simulink model "adaptivePID"  (R2024a)
settings: Solver=ode4  StartTime=0.0  StopTime=5  FixedStep=1E-5  RelTol=1e-3
values from neighbouring files (symbols this model uses):
  initial_1 =     [ma.mat]    (also in regulation.mat)
  observer =     [ma.mat]    (also in regulation.mat)
  sliding =     [regulation.mat]
  x = [input(1);input(2);input(3)]    [Dist_observer.m]    (also in is501nmtbModel_simu.m; is501nmtbModel_simu1.m; ma.mat = ; neuronalPID.m = entr(4))
  y = [input(7),input(8),input(9)]'    [estimator.m]    (also in is501nmtbModel_simu1.m = B * x + Td; ma.mat = ; regulation.mat = )
  z =     [ma.mat]    (also in regulation.mat)
settings Model: Creator=b_ant  LastModifiedBy=b_ant
settings SolverCC: ZeroCrossAlgorithm=Adaptive
settings DebuggingCC: IgnoredZcDiagnostic=none  UnconnectedInputMsg=warning  UnconnectedOutputMsg=warning  UnconnectedLineMsg=warning
settings ModelReferenceCC: EnableRefExpFcnMdlSchedulingChecks=on
settings RTWCC: GPUComputeCapability=3.5  DLArmComputeVersion=19.05

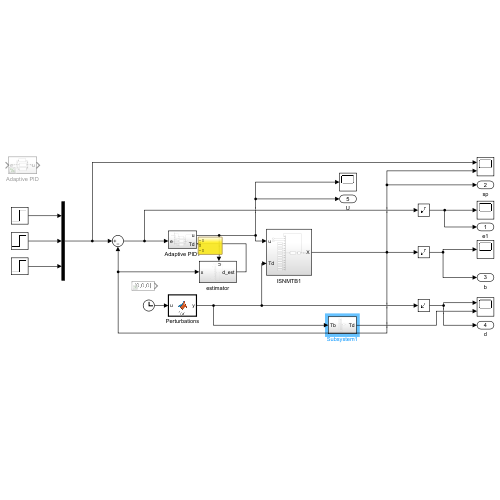
[thumbnail: Simulink's stored preview of the top-level diagram]
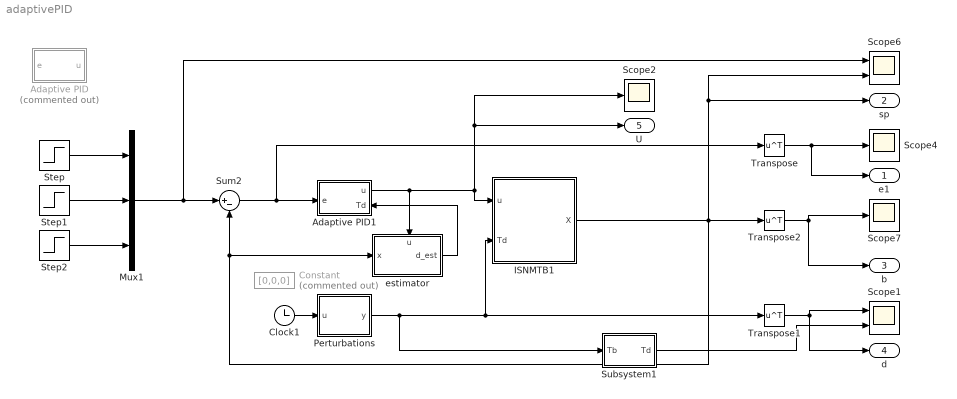
== system adaptivePID ==
  Adaptive PID : Subsystem  Commented=on
  Adaptive PID1 : Subsystem
      settings: PortSchema="{\"entries\":[{\"content\":{\"sides\":[{\"content\":{\"connectorIds\":[\"In1\"]},\"type\":\"ConnectorPlacement.EquallySpacedRectSide\",\"uuid\":\"d8958802-6b7a-44a5-a52a-ddab063e146c\"},{\"content\":{\"connectorIds\":[\"Out1\",\"In2\"],\"side\":\"RIGHT\"},\"type\":\"ConnectorPlacement.EquallySpacedRectSide\",\"uuid\":\"da9beaf8-944d-47f3-af69-928c263140b5\"},{\"content\":{\"side\":\"TOP\"},\"type\":\"ConnectorPlacement.EquallySpacedRectSide\",\"uuid\":\"6b1d50a8-02e3-44c8-b40e-0b40ffb17dcd\"}]},\"type\":\"ConnectorPlacement.EquallySpacedConnector\",\"uuid\":\"8706e551-040c-4dd8-82c5-a7bc820e0e37\"}],\"packageUris\":[\"http://schema.mathworks.com/mf0/Connector/R2020b\"],\"version\":\"1.0\"}"
  Clock1 : Clock
      settings: Decimation=1000
  Constant : Constant  Commented=on  Value=[0,0,0]
  ISNMTB1 : Subsystem
  Mux1 : Mux  Inputs=3
  Perturbations : MATLAB Function  TreatAsAtomicUnit=on
  Scope1 : Scope  NumInputPorts=2
  Scope2 : Scope
  Scope4 : Scope
  Scope6 : Scope  NumInputPorts=2
  Scope7 : Scope
  Step : Step  Time=0.1  SampleTime=0
  Step1 : Step  Time=0.1  SampleTime=0
  Step2 : Step  Time=0.1  After=0.1  SampleTime=0
  Subsystem1 : Subsystem
  Sum2 : Sum  Inputs=|+-
  Transpose : Math  Operator=transpose
  Transpose1 : Math  Operator=transpose
  Transpose2 : Math  Operator=transpose
  estimator : Subsystem
      settings: PortSchema="{\"entries\":[{\"content\":{\"sides\":[{\"content\":{\"connectorIds\":[\"In1\"]},\"type\":\"ConnectorPlacement.EquallySpacedRectSide\",\"uuid\":\"f9e844d6-ee13-4ae8-8d73-084dc6b9c230\"},{\"content\":{\"connectorIds\":[\"Out1\"],\"side\":\"RIGHT\"},\"type\":\"ConnectorPlacement.EquallySpacedRectSide\",\"uuid\":\"c081e574-2129-4344-8b67-56cd55c23b50\"},{\"content\":{\"connectorIds\":[\"In2\"],\"side\":\"TOP\"},\"type\":\"ConnectorPlacement.EquallySpacedRectSide\",\"uuid\":\"bf6f2985-e51e-41d0-a8b1-b5505659e5f3\"},{\"content\":{\"side\":\"BOTTOM\"},\"type\":\"ConnectorPlacement.EquallySpacedRectSide\",\"uuid\":\"e1697b77-960b-449d-843b-5909cf972339\"}]},\"type\":\"ConnectorPlacement.EquallySpacedConnector\",\"uuid\":\"c9da1c41-5311-41bf-ab5b-06506202d90f\"}],\"packageUris\":[\"http://schema.mathworks.com/mf0/Connector/R2020b\"],\"version\":\"1.0\"}"
  e1 : Outport
  sp : Outport  Port=2
  b : Outport  Port=3
  d : Outport  Port=4
  U : Outport  Port=5
  wires:
  Transpose1/1 -> Scope1/1, d/1
  ISNMTB1/1(X) -> sp/1, Scope6/2, estimator/1(x), Sum2/2, Transpose2/1
  Sum2/1 -> Transpose/1, Adaptive PID1/1(e)
  Step2/1 -> Mux1/3
  Transpose2/1 -> Scope7/1, b/1
  Step1/1 -> Mux1/2
  Clock1/1 -> Perturbations/1(u)
  Transpose/1 -> e1/1, Scope4/1
  Step/1 -> Mux1/1
  Mux1/1 -> Sum2/1, Scope6/1
  Adaptive PID1/1(u) -> estimator/2(u), ISNMTB1/1(u), U/1, Scope2/1
  estimator/1(d_est) -> Adaptive PID1/2(Td)
  Subsystem1/1(Td) -> Scope1/2
  Perturbations/1(y) -> ISNMTB1/2(Td), Transpose1/1, Subsystem1/1(Tb)

== system adaptivePID/Adaptive PID ==
  e : Inport
  Demux1 : Demux  Outputs=3
  Mux : Mux  Inputs=3
  x controller : Subsystem
  y controller : Subsystem
  z controller : Subsystem
  u : Outport
  wires:
  z controller/1(u) -> Mux/3
  Demux1/2 -> y controller/1(e)
  x controller/1(u) -> Mux/1
  e/1 -> Demux1/1
  y controller/1(u) -> Mux/2
  Demux1/3 -> z controller/1(e)
  Demux1/1 -> x controller/1(e)
  Mux/1 -> u/1

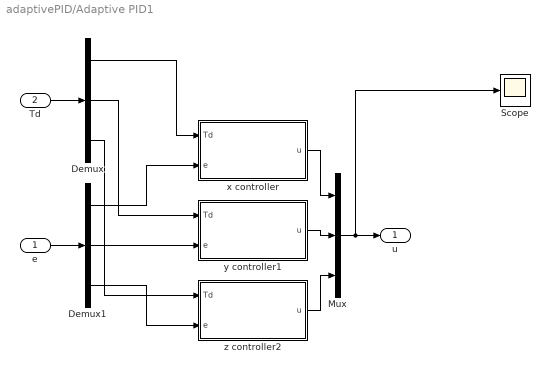
== system adaptivePID/Adaptive PID1 ==
  e : Inport
  Td : Inport  Port=2
  Demux : Demux  Outputs=3
  Demux1 : Demux  Outputs=3
  Mux : Mux  Inputs=3
  Scope : Scope
  x controller : Subsystem
  y controller1 : Subsystem
  z controller2 : Subsystem
  u : Outport
  wires:
  Demux1/2 -> y controller1/2(e)
  x controller/1(u) -> Mux/1
  e/1 -> Demux1/1
  Demux1/1 -> x controller/2(e)
  Mux/1 -> Scope/1, u/1
  Demux1/3 -> z controller2/2(e)
  Demux/3 -> z controller2/1(Td)
  Demux/2 -> y controller1/1(Td)
  Demux/1 -> x controller/1(Td)
  Td/1 -> Demux/1
  y controller1/1(u) -> Mux/2
  z controller2/1(u) -> Mux/3

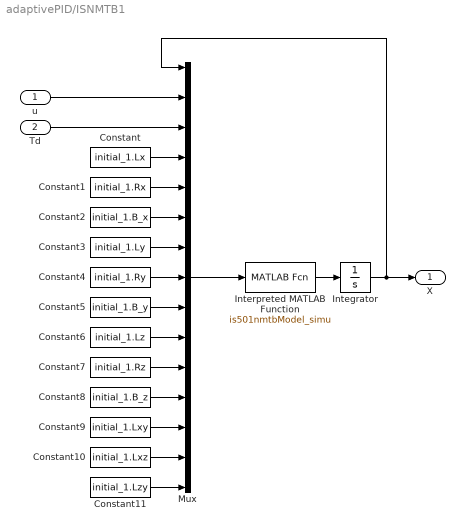
== system adaptivePID/ISNMTB1 ==
  u : Inport
  Td : Inport  Port=2
  Constant : Constant  Value=initial_1.Lx
  Constant1 : Constant  Value=initial_1.Rx
  Constant10 : Constant  Value=initial_1.Lxz
  Constant11 : Constant  Value=initial_1.Lzy
  Constant2 : Constant  Value=initial_1.B_x
  Constant3 : Constant  Value=initial_1.Ly
  Constant4 : Constant  Value=initial_1.Ry
  Constant5 : Constant  Value=initial_1.B_y
  Constant6 : Constant  Value=initial_1.Lz
  Constant7 : Constant  Value=initial_1.Rz
  Constant8 : Constant  Value=initial_1.B_z
  Constant9 : Constant  Value=initial_1.Lxy
  Integrator : Integrator  InitialCondition=[3.249E4, -2.265E4, 3.655E4]
  Interpreted MATLAB Function : MATLABFcn  MATLABFcn=is501nmtbModel_simu
  Mux : Mux  Inputs=15
  X : Outport
  wires:
  Interpreted MATLAB Function/1 -> Integrator/1
  Integrator/1 -> X/1, Mux/1
  Mux/1 -> Interpreted MATLAB Function/1
  u/1 -> Mux/2
  Td/1 -> Mux/3
  Constant/1 -> Mux/4
  Constant1/1 -> Mux/5
  Constant2/1 -> Mux/6
  Constant3/1 -> Mux/7
  Constant4/1 -> Mux/8
  Constant5/1 -> Mux/9
  Constant6/1 -> Mux/10
  Constant7/1 -> Mux/11
  Constant8/1 -> Mux/12
  Constant9/1 -> Mux/13
  Constant10/1 -> Mux/14
  Constant11/1 -> Mux/15

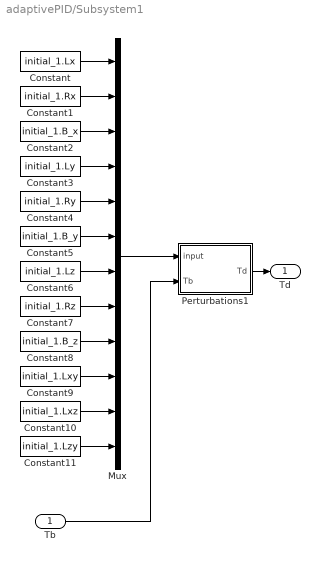
== system adaptivePID/Subsystem1 ==
  Tb : Inport
  Constant : Constant  Value=initial_1.Lx
  Constant1 : Constant  Value=initial_1.Rx
  Constant10 : Constant  Value=initial_1.Lxz
  Constant11 : Constant  Value=initial_1.Lzy
  Constant2 : Constant  Value=initial_1.B_x
  Constant3 : Constant  Value=initial_1.Ly
  Constant4 : Constant  Value=initial_1.Ry
  Constant5 : Constant  Value=initial_1.B_y
  Constant6 : Constant  Value=initial_1.Lz
  Constant7 : Constant  Value=initial_1.Rz
  Constant8 : Constant  Value=initial_1.B_z
  Constant9 : Constant  Value=initial_1.Lxy
  Mux : Mux  Inputs=12
  Perturbations1 : MATLAB Function  TreatAsAtomicUnit=on
  Td : Outport
  wires:
  Constant2/1 -> Mux/3
  Constant6/1 -> Mux/7
  Constant7/1 -> Mux/8
  Constant8/1 -> Mux/9
  Constant9/1 -> Mux/10
  Constant/1 -> Mux/1
  Constant11/1 -> Mux/12
  Constant10/1 -> Mux/11
  Constant5/1 -> Mux/6
  Constant3/1 -> Mux/4
  Mux/1 -> Perturbations1/1(input)
  Constant1/1 -> Mux/2
  Constant4/1 -> Mux/5
  Tb/1 -> Perturbations1/2(Tb)
  Perturbations1/1(Td) -> Td/1

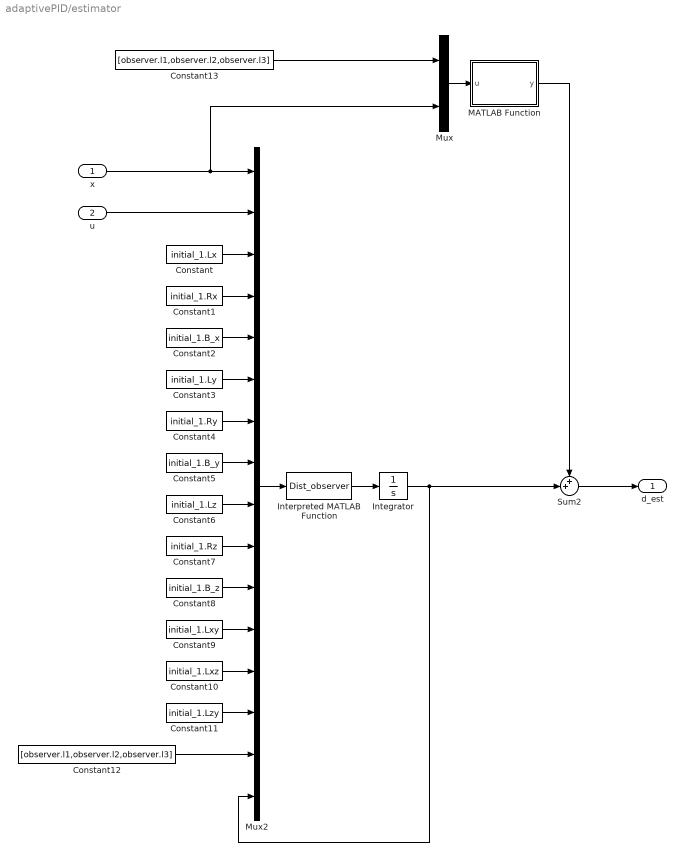
== system adaptivePID/estimator ==
  x : Inport
  u : Inport  Port=2
  Constant : Constant  Value=initial_1.Lx
  Constant1 : Constant  Value=initial_1.Rx
  Constant10 : Constant  Value=initial_1.Lxz
  Constant11 : Constant  Value=initial_1.Lzy
  Constant12 : Constant  Value=[observer.l1,observer.l2,observer.l3]
  Constant13 : Constant  Value=[observer.l1,observer.l2,observer.l3]
  Constant2 : Constant  Value=initial_1.B_x
  Constant3 : Constant  Value=initial_1.Ly
  Constant4 : Constant  Value=initial_1.Ry
  Constant5 : Constant  Value=initial_1.B_y
  Constant6 : Constant  Value=initial_1.Lz
  Constant7 : Constant  Value=initial_1.Rz
  Constant8 : Constant  Value=initial_1.B_z
  Constant9 : Constant  Value=initial_1.Lxy
  Integrator : Integrator  InitialCondition=[0,0,0]
  Interpreted MATLAB Function : MATLABFcn  MATLABFcn=Dist_observer
  MATLAB Function : MATLAB Function  TreatAsAtomicUnit=on
  Mux : Mux  Inputs=2
  Mux2 : Mux  Inputs=16
  Sum2 : Sum  Inputs=++|
  d_est : Outport
  wires:
  Constant6/1 -> Mux2/9
  MATLAB Function/1(y) -> Sum2/1
  Constant10/1 -> Mux2/13
  Integrator/1 -> Sum2/2, Mux2/16
  Interpreted MATLAB Function/1 -> Integrator/1
  Constant2/1 -> Mux2/5
  Constant4/1 -> Mux2/7
  Constant7/1 -> Mux2/10
  Mux2/1 -> Interpreted MATLAB Function/1
  Constant11/1 -> Mux2/14
  Constant8/1 -> Mux2/11
  Constant1/1 -> Mux2/4
  Constant3/1 -> Mux2/6
  Constant/1 -> Mux2/3
  Constant9/1 -> Mux2/12
  Constant5/1 -> Mux2/8
  Constant12/1 -> Mux2/15
  u/1 -> Mux2/2
  Sum2/1 -> d_est/1
  Constant13/1 -> Mux/1
  Mux/1 -> MATLAB Function/1(u)
  x/1 -> Mux/2, Mux2/1

== system adaptivePID/Adaptive PID/x controller ==
  e : Inport
  Adaptation Law : Subsystem  mask{alpha=x.alpha, beta=x.beta, epsilon=x.epsilon, n=x.n, kd0=x.kd_init, ki0=x.ki_init, kp0=x.kp_init}
      mask prompts: kd0 "kd_0:"; ki0 "ki_0:"; kp0 "kp_0:"
      mask TypeOptions alpha: alpha/Value
      mask TypeOptions beta: beta/Value
      mask TypeOptions epsilon: epsilon/Value
      mask TypeOptions n: n/Value
      mask TypeOptions kd0: kd0/Value
      mask TypeOptions ki0: ki0/Value
      mask TypeOptions kp0: kp0/Value
  PID controller : Subsystem
  Scope : Scope
  Sliding surface : Subsystem  mask{Gain=x.lambda}
      mask prompts: Gain "Simulink:blkprm_prompts:GainGain"
      mask TypeOptions Gain: Gain/Gain
      mask DialogControl Gain Prompt: Gain:
  error subsystem : Subsystem
  u : Outport
  wires:
  Sliding surface/1(s) -> Adaptation Law/2(s)
  Sliding surface/2(s_dot) -> Adaptation Law/3(s_dot)
  PID controller/1(u) -> u/1
  error subsystem/1(MyPi) -> PID controller/2(MyPi), Adaptation Law/1(myPi)
  e/1 -> Sliding surface/1(e), error subsystem/1(e)
  Adaptation Law/1(theta) -> Scope/1, PID controller/1(theta)

== system adaptivePID/Adaptive PID/y controller ==
  e : Inport
  Adaptation Law : Subsystem  mask{alpha=y.alpha, beta=y.beta, epsilon=y.epsilon, n=y.n, kd0=y.kd_init, ki0=y.ki_init, kp0=y.kp_init}
      mask prompts: kd0 "kd_0:"; ki0 "ki_0:"; kp0 "kp_0:"
      mask TypeOptions alpha: alpha/Value
      mask TypeOptions beta: beta/Value
      mask TypeOptions epsilon: epsilon/Value
      mask TypeOptions n: n/Value
      mask TypeOptions kd0: kd0/Value
      mask TypeOptions ki0: ki0/Value
      mask TypeOptions kp0: kp0/Value
  PID controller : Subsystem
  Scope : Scope
  Sliding surface : Subsystem  mask{Gain=y.lambda}
      mask prompts: Gain "Simulink:blkprm_prompts:GainGain"
      mask TypeOptions Gain: Gain/Gain
      mask DialogControl Gain Prompt: Gain:
  error subsystem : Subsystem
  u : Outport
  wires:
  e/1 -> Sliding surface/1(e), error subsystem/1(e)
  error subsystem/1(MyPi) -> Adaptation Law/1(myPi), PID controller/2(MyPi)
  Adaptation Law/1(theta) -> PID controller/1(theta), Scope/1
  PID controller/1(u) -> u/1
  Sliding surface/2(s_dot) -> Adaptation Law/3(s_dot)
  Sliding surface/1(s) -> Adaptation Law/2(s)

== system adaptivePID/Adaptive PID/z controller ==
  e : Inport
  Adaptation Law : Subsystem  mask{alpha=z.alpha, beta=z.beta, epsilon=z.epsilon, n=z.n, kd0=z.kd_init, ki0=z.ki_init, kp0=z.kp_init}
      mask prompts: kd0 "kd_0:"; ki0 "ki_0:"; kp0 "kp_0:"
      mask TypeOptions alpha: alpha/Value
      mask TypeOptions beta: beta/Value
      mask TypeOptions epsilon: epsilon/Value
      mask TypeOptions n: n/Value
      mask TypeOptions kd0: kd0/Value
      mask TypeOptions ki0: ki0/Value
      mask TypeOptions kp0: kp0/Value
  PID controller : Subsystem
  Scope : Scope
  Sliding surface : Subsystem  mask{Gain=z.lambda}
      mask prompts: Gain "Simulink:blkprm_prompts:GainGain"
      mask TypeOptions Gain: Gain/Gain
      mask DialogControl Gain Prompt: Gain:
  error subsystem : Subsystem
  u : Outport
  wires:
  Sliding surface/1(s) -> Adaptation Law/2(s)
  Sliding surface/2(s_dot) -> Adaptation Law/3(s_dot)
  PID controller/1(u) -> u/1
  Adaptation Law/1(theta) -> Scope/1, PID controller/1(theta)
  error subsystem/1(MyPi) -> PID controller/2(MyPi), Adaptation Law/1(myPi)
  e/1 -> error subsystem/1(e), Sliding surface/1(e)

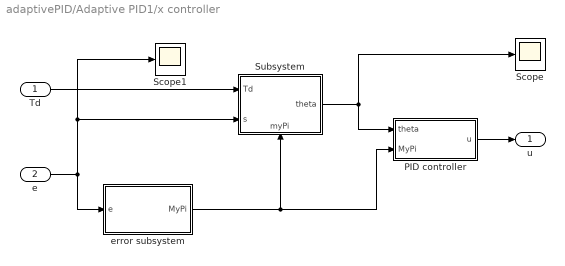
== system adaptivePID/Adaptive PID1/x controller ==
  Td : Inport
  e : Inport  Port=2
  PID controller : Subsystem
  Scope : Scope
  Scope1 : Scope
  Subsystem : Subsystem
      settings: PortSchema="{\"entries\":[{\"content\":{\"sides\":[{\"content\":{\"connectorIds\":[\"In1\",\"In2\"]},\"type\":\"ConnectorPlacement.EquallySpacedRectSide\",\"uuid\":\"240bad6f-f804-428c-a3a0-dcf6f9934484\"},{\"content\":{\"connectorIds\":[\"Out1\"],\"side\":\"RIGHT\"},\"type\":\"ConnectorPlacement.EquallySpacedRectSide\",\"uuid\":\"1a0c794f-cbf7-475a-a374-9465cebda297\"},{\"content\":{\"side\":\"TOP\"},\"type\":\"ConnectorPlacement.EquallySpacedRectSide\",\"uuid\":\"3b98e4f4-718b-47e5-85a1-a51970b349c9\"},{\"content\":{\"connectorIds\":[\"In3\"],\"side\":\"BOTTOM\"},\"type\":\"ConnectorPlacement.EquallySpacedRectSide\",\"uuid\":\"519e2597-1479-45b2-9e81-d744a6fccd79\"}]},\"type\":\"ConnectorPlacement.EquallySpacedConnector\",\"uuid\":\"08a721e1-b25b-470b-a637-c1c50488aa37\"}],\"packageUris\":[\"http://schema.mathworks.com/mf0/Connector/R2020b\"],\"version\":\"1.0\"}"
  error subsystem : Subsystem
  u : Outport
  wires:
  PID controller/1(u) -> u/1
  error subsystem/1(MyPi) -> Subsystem/3(myPi), PID controller/2(MyPi)
  e/1 -> error subsystem/1(e), Scope1/1, Subsystem/2(s)
  Subsystem/1(theta) -> Scope/1, PID controller/1(theta)
  Td/1 -> Subsystem/1(Td)

== system adaptivePID/Adaptive PID1/y controller1 ==
  Td : Inport
  e : Inport  Port=2
  PID controller : Subsystem
  Scope : Scope
  Subsystem : Subsystem
      settings: PortSchema="{\"entries\":[{\"content\":{\"sides\":[{\"content\":{\"connectorIds\":[\"In1\",\"In2\"]},\"type\":\"ConnectorPlacement.EquallySpacedRectSide\",\"uuid\":\"240bad6f-f804-428c-a3a0-dcf6f9934484\"},{\"content\":{\"connectorIds\":[\"Out1\"],\"side\":\"RIGHT\"},\"type\":\"ConnectorPlacement.EquallySpacedRectSide\",\"uuid\":\"1a0c794f-cbf7-475a-a374-9465cebda297\"},{\"content\":{\"side\":\"TOP\"},\"type\":\"ConnectorPlacement.EquallySpacedRectSide\",\"uuid\":\"3b98e4f4-718b-47e5-85a1-a51970b349c9\"},{\"content\":{\"connectorIds\":[\"In3\"],\"side\":\"BOTTOM\"},\"type\":\"ConnectorPlacement.EquallySpacedRectSide\",\"uuid\":\"519e2597-1479-45b2-9e81-d744a6fccd79\"}]},\"type\":\"ConnectorPlacement.EquallySpacedConnector\",\"uuid\":\"08a721e1-b25b-470b-a637-c1c50488aa37\"}],\"packageUris\":[\"http://schema.mathworks.com/mf0/Connector/R2020b\"],\"version\":\"1.0\"}"
  error subsystem : Subsystem
  u : Outport
  wires:
  PID controller/1(u) -> u/1
  error subsystem/1(MyPi) -> Subsystem/3(myPi), PID controller/2(MyPi)
  e/1 -> error subsystem/1(e), Subsystem/2(s)
  Subsystem/1(theta) -> Scope/1, PID controller/1(theta)
  Td/1 -> Subsystem/1(Td)

== system adaptivePID/Adaptive PID1/z controller2 ==
  Td : Inport
  e : Inport  Port=2
  PID controller : Subsystem
  Scope : Scope
  Subsystem : Subsystem
      settings: PortSchema="{\"entries\":[{\"content\":{\"sides\":[{\"content\":{\"connectorIds\":[\"In1\",\"In2\"]},\"type\":\"ConnectorPlacement.EquallySpacedRectSide\",\"uuid\":\"240bad6f-f804-428c-a3a0-dcf6f9934484\"},{\"content\":{\"connectorIds\":[\"Out1\"],\"side\":\"RIGHT\"},\"type\":\"ConnectorPlacement.EquallySpacedRectSide\",\"uuid\":\"1a0c794f-cbf7-475a-a374-9465cebda297\"},{\"content\":{\"side\":\"TOP\"},\"type\":\"ConnectorPlacement.EquallySpacedRectSide\",\"uuid\":\"3b98e4f4-718b-47e5-85a1-a51970b349c9\"},{\"content\":{\"connectorIds\":[\"In3\"],\"side\":\"BOTTOM\"},\"type\":\"ConnectorPlacement.EquallySpacedRectSide\",\"uuid\":\"519e2597-1479-45b2-9e81-d744a6fccd79\"}]},\"type\":\"ConnectorPlacement.EquallySpacedConnector\",\"uuid\":\"08a721e1-b25b-470b-a637-c1c50488aa37\"}],\"packageUris\":[\"http://schema.mathworks.com/mf0/Connector/R2020b\"],\"version\":\"1.0\"}"
  error subsystem : Subsystem
  u : Outport
  wires:
  PID controller/1(u) -> u/1
  error subsystem/1(MyPi) -> Subsystem/3(myPi), PID controller/2(MyPi)
  e/1 -> error subsystem/1(e), Subsystem/2(s)
  Subsystem/1(theta) -> Scope/1, PID controller/1(theta)
  Td/1 -> Subsystem/1(Td)

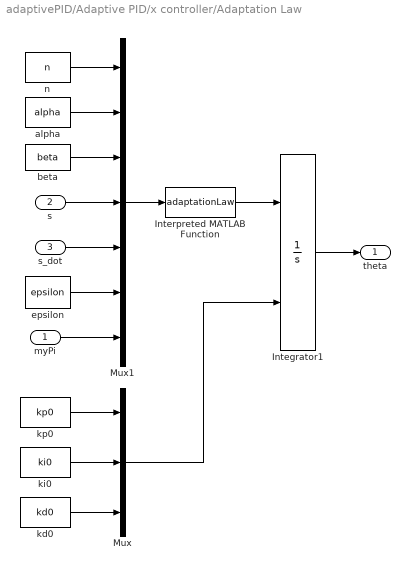
== system adaptivePID/Adaptive PID/x controller/Adaptation Law ==
  myPi : Inport
  s : Inport  Port=2
  s_dot : Inport  Port=3
  Integrator1 : Integrator  InitialConditionSource=external  InitialCondition=[1.460477259865257e-04,6.548069875818259e-05,0]
  Interpreted MATLAB Function : MATLABFcn  MATLABFcn=adaptationLaw
  Mux : Mux  Inputs=3
  Mux1 : Mux  Inputs=7
  alpha : Constant  Value=alpha
  beta : Constant  Value=beta
  epsilon : Constant  Value=epsilon
  kd0 : Constant  Value=kd0
  ki0 : Constant  Value=ki0
  kp0 : Constant  Value=kp0
  n : Constant  Value=n
  theta : Outport
  wires:
  alpha/1 -> Mux1/2
  Interpreted MATLAB Function/1 -> Integrator1/1
  myPi/1 -> Mux1/7
  s/1 -> Mux1/4
  epsilon/1 -> Mux1/6
  Integrator1/1 -> theta/1
  s_dot/1 -> Mux1/5
  beta/1 -> Mux1/3
  Mux1/1 -> Interpreted MATLAB Function/1
  n/1 -> Mux1/1
  ki0/1 -> Mux/2
  Mux/1 -> Integrator1/2
  kp0/1 -> Mux/1
  kd0/1 -> Mux/3

== system adaptivePID/Adaptive PID/x controller/PID controller ==
  theta : Inport
  MyPi : Inport  Port=2
  Interpreted MATLAB Function1 : MATLABFcn  MATLABFcn=controlLaw  OutputDimensions=1
  Mux2 : Mux  Inputs=2
  u : Outport
  wires:
  Mux2/1 -> Interpreted MATLAB Function1/1
  theta/1 -> Mux2/1
  Interpreted MATLAB Function1/1 -> u/1
  MyPi/1 -> Mux2/2

== system adaptivePID/Adaptive PID/x controller/Sliding surface ==
  note: s
  note: e
  e : Inport
  Add : Sum
  Derivative : Derivative
  Derivative1 : Derivative
  Gain : Gain  Gain=Gain
  s : Outport
  s_dot : Outport  Port=2
  wires:
  Add/1 -> s/1, Derivative/1
  Gain/1 -> Add/1
  e/1 -> Derivative1/1, Gain/1
  Derivative1/1 -> Add/2
  Derivative/1 -> s_dot/1

== system adaptivePID/Adaptive PID/x controller/error subsystem ==
  e : Inport
  Derivative : Derivative
  Integrator : Integrator
  Mux : Mux  Inputs=3
  MyPi : Outport
  wires:
  e/1 -> Derivative/1, Mux/1, Integrator/1
  Integrator/1 -> Mux/2
  Mux/1 -> MyPi/1
  Derivative/1 -> Mux/3

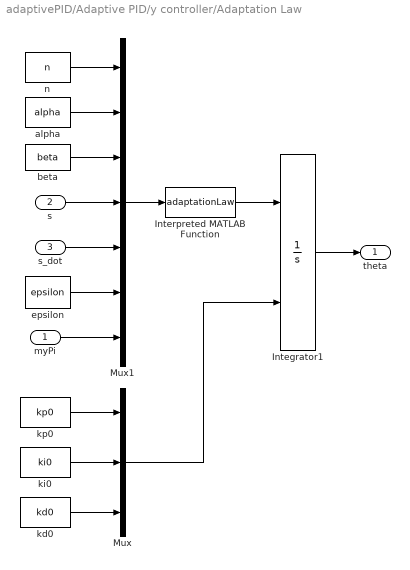
== system adaptivePID/Adaptive PID/y controller/Adaptation Law ==
  myPi : Inport
  s : Inport  Port=2
  s_dot : Inport  Port=3
  Integrator1 : Integrator  InitialConditionSource=external  InitialCondition=[1.460477259865257e-04,6.548069875818259e-05,0]
  Interpreted MATLAB Function : MATLABFcn  MATLABFcn=adaptationLaw
  Mux : Mux  Inputs=3
  Mux1 : Mux  Inputs=7
  alpha : Constant  Value=alpha
  beta : Constant  Value=beta
  epsilon : Constant  Value=epsilon
  kd0 : Constant  Value=kd0
  ki0 : Constant  Value=ki0
  kp0 : Constant  Value=kp0
  n : Constant  Value=n
  theta : Outport
  wires:
  kd0/1 -> Mux/3
  kp0/1 -> Mux/1
  Mux/1 -> Integrator1/2
  ki0/1 -> Mux/2
  n/1 -> Mux1/1
  Mux1/1 -> Interpreted MATLAB Function/1
  beta/1 -> Mux1/3
  s_dot/1 -> Mux1/5
  Integrator1/1 -> theta/1
  epsilon/1 -> Mux1/6
  s/1 -> Mux1/4
  myPi/1 -> Mux1/7
  Interpreted MATLAB Function/1 -> Integrator1/1
  alpha/1 -> Mux1/2

== system adaptivePID/Adaptive PID/y controller/PID controller ==
  theta : Inport
  MyPi : Inport  Port=2
  Interpreted MATLAB Function1 : MATLABFcn  MATLABFcn=controlLaw  OutputDimensions=1
  Mux2 : Mux  Inputs=2
  u : Outport
  wires:
  MyPi/1 -> Mux2/2
  Interpreted MATLAB Function1/1 -> u/1
  theta/1 -> Mux2/1
  Mux2/1 -> Interpreted MATLAB Function1/1

== system adaptivePID/Adaptive PID/y controller/Sliding surface ==
  note: e
  note: s
  e : Inport
  Add : Sum
  Derivative : Derivative
  Derivative1 : Derivative
  Gain : Gain  Gain=Gain
  s : Outport
  s_dot : Outport  Port=2
  wires:
  Derivative/1 -> s_dot/1
  Derivative1/1 -> Add/2
  e/1 -> Derivative1/1, Gain/1
  Gain/1 -> Add/1
  Add/1 -> s/1, Derivative/1

== system adaptivePID/Adaptive PID/y controller/error subsystem ==
  e : Inport
  Derivative : Derivative
  Integrator : Integrator
  Mux : Mux  Inputs=3
  MyPi : Outport
  wires:
  Derivative/1 -> Mux/3
  Mux/1 -> MyPi/1
  Integrator/1 -> Mux/2
  e/1 -> Derivative/1, Integrator/1, Mux/1

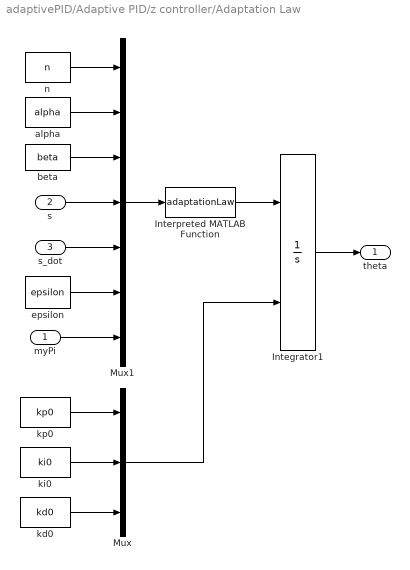
== system adaptivePID/Adaptive PID/z controller/Adaptation Law ==
  myPi : Inport
  s : Inport  Port=2
  s_dot : Inport  Port=3
  Integrator1 : Integrator  InitialConditionSource=external  InitialCondition=[1.460477259865257e-04,6.548069875818259e-05,0]
  Interpreted MATLAB Function : MATLABFcn  MATLABFcn=adaptationLaw
  Mux : Mux  Inputs=3
  Mux1 : Mux  Inputs=7
  alpha : Constant  Value=alpha
  beta : Constant  Value=beta
  epsilon : Constant  Value=epsilon
  kd0 : Constant  Value=kd0
  ki0 : Constant  Value=ki0
  kp0 : Constant  Value=kp0
  n : Constant  Value=n
  theta : Outport
  wires:
  alpha/1 -> Mux1/2
  Interpreted MATLAB Function/1 -> Integrator1/1
  myPi/1 -> Mux1/7
  s/1 -> Mux1/4
  epsilon/1 -> Mux1/6
  Integrator1/1 -> theta/1
  s_dot/1 -> Mux1/5
  beta/1 -> Mux1/3
  Mux1/1 -> Interpreted MATLAB Function/1
  n/1 -> Mux1/1
  ki0/1 -> Mux/2
  Mux/1 -> Integrator1/2
  kp0/1 -> Mux/1
  kd0/1 -> Mux/3

== system adaptivePID/Adaptive PID/z controller/PID controller ==
  theta : Inport
  MyPi : Inport  Port=2
  Interpreted MATLAB Function1 : MATLABFcn  MATLABFcn=controlLaw  OutputDimensions=1
  Mux2 : Mux  Inputs=2
  u : Outport
  wires:
  Mux2/1 -> Interpreted MATLAB Function1/1
  theta/1 -> Mux2/1
  Interpreted MATLAB Function1/1 -> u/1
  MyPi/1 -> Mux2/2

== system adaptivePID/Adaptive PID/z controller/Sliding surface ==
  note: s
  note: e
  e : Inport
  Add : Sum
  Derivative : Derivative
  Derivative1 : Derivative
  Gain : Gain  Gain=Gain
  s : Outport
  s_dot : Outport  Port=2
  wires:
  Add/1 -> s/1, Derivative/1
  Gain/1 -> Add/1
  e/1 -> Derivative1/1, Gain/1
  Derivative1/1 -> Add/2
  Derivative/1 -> s_dot/1

== system adaptivePID/Adaptive PID/z controller/error subsystem ==
  e : Inport
  Derivative : Derivative
  Integrator : Integrator
  Mux : Mux  Inputs=3
  MyPi : Outport
  wires:
  e/1 -> Derivative/1, Mux/1, Integrator/1
  Integrator/1 -> Mux/2
  Mux/1 -> MyPi/1
  Derivative/1 -> Mux/3

== system adaptivePID/Adaptive PID1/x controller/PID controller ==
  theta : Inport
  MyPi : Inport  Port=2
  Interpreted MATLAB Function1 : MATLABFcn  MATLABFcn=controlLaw  OutputDimensions=1
  Mux2 : Mux  Inputs=2
  u : Outport
  wires:
  Mux2/1 -> Interpreted MATLAB Function1/1
  theta/1 -> Mux2/1
  Interpreted MATLAB Function1/1 -> u/1
  MyPi/1 -> Mux2/2

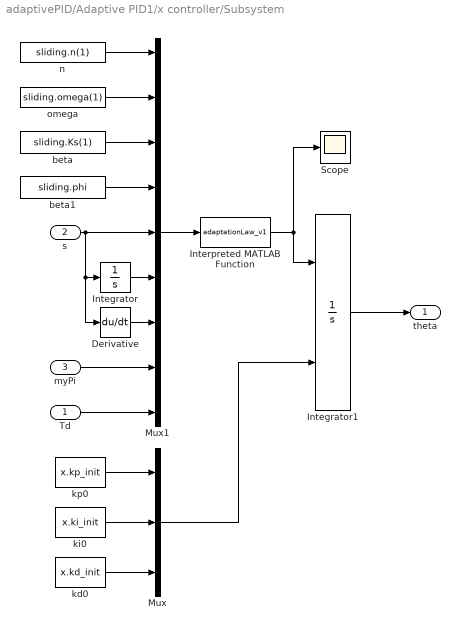
== system adaptivePID/Adaptive PID1/x controller/Subsystem ==
  Td : Inport
  s : Inport  Port=2
  myPi : Inport  Port=3
  Derivative : Derivative
  Integrator : Integrator
  Integrator1 : Integrator  InitialConditionSource=external  InitialCondition=[1.460477259865257e-04,6.548069875818259e-05,0]
  Interpreted MATLAB Function : MATLABFcn  MATLABFcn=adaptationLaw_v1
  Mux : Mux  Inputs=3
  Mux1 : Mux  Inputs=9
  Scope : Scope
  beta : Constant  Value=sliding.Ks(1)
  beta1 : Constant  Value=sliding.phi
  kd0 : Constant  Value=x.kd_init
  ki0 : Constant  Value=x.ki_init
  kp0 : Constant  Value=x.kp_init
  n : Constant  Value=sliding.n(1)
  omega : Constant  Value=sliding.omega(1)
  theta : Outport
  wires:
  beta/1 -> Mux1/3
  n/1 -> Mux1/1
  kd0/1 -> Mux/3
  kp0/1 -> Mux/1
  ki0/1 -> Mux/2
  Integrator1/1 -> theta/1
  omega/1 -> Mux1/2
  Mux1/1 -> Interpreted MATLAB Function/1
  Mux/1 -> Integrator1/2
  Interpreted MATLAB Function/1 -> Integrator1/1, Scope/1
  beta1/1 -> Mux1/4
  Integrator/1 -> Mux1/6
  s/1 -> Mux1/5, Derivative/1, Integrator/1
  Derivative/1 -> Mux1/7
  myPi/1 -> Mux1/8
  Td/1 -> Mux1/9

== system adaptivePID/Adaptive PID1/x controller/error subsystem ==
  e : Inport
  Derivative : Derivative
  Integrator : Integrator
  Mux : Mux  Inputs=3
  MyPi : Outport
  wires:
  e/1 -> Derivative/1, Mux/1, Integrator/1
  Integrator/1 -> Mux/2
  Mux/1 -> MyPi/1
  Derivative/1 -> Mux/3

== system adaptivePID/Adaptive PID1/y controller1/PID controller ==
  theta : Inport
  MyPi : Inport  Port=2
  Interpreted MATLAB Function1 : MATLABFcn  MATLABFcn=controlLaw  OutputDimensions=1
  Mux2 : Mux  Inputs=2
  u : Outport
  wires:
  Mux2/1 -> Interpreted MATLAB Function1/1
  theta/1 -> Mux2/1
  Interpreted MATLAB Function1/1 -> u/1
  MyPi/1 -> Mux2/2

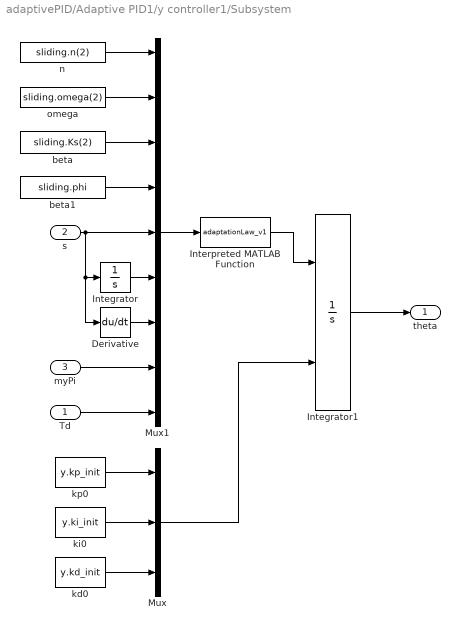
== system adaptivePID/Adaptive PID1/y controller1/Subsystem ==
  Td : Inport
  s : Inport  Port=2
  myPi : Inport  Port=3
  Derivative : Derivative
  Integrator : Integrator
  Integrator1 : Integrator  InitialConditionSource=external  InitialCondition=[1.460477259865257e-04,6.548069875818259e-05,0]
  Interpreted MATLAB Function : MATLABFcn  MATLABFcn=adaptationLaw_v1
  Mux : Mux  Inputs=3
  Mux1 : Mux  Inputs=9
  beta : Constant  Value=sliding.Ks(2)
  beta1 : Constant  Value=sliding.phi
  kd0 : Constant  Value=y.kd_init
  ki0 : Constant  Value=y.ki_init
  kp0 : Constant  Value=y.kp_init
  n : Constant  Value=sliding.n(2)
  omega : Constant  Value=sliding.omega(2)
  theta : Outport
  wires:
  beta/1 -> Mux1/3
  n/1 -> Mux1/1
  kd0/1 -> Mux/3
  kp0/1 -> Mux/1
  ki0/1 -> Mux/2
  Integrator1/1 -> theta/1
  omega/1 -> Mux1/2
  Mux1/1 -> Interpreted MATLAB Function/1
  Mux/1 -> Integrator1/2
  Interpreted MATLAB Function/1 -> Integrator1/1
  beta1/1 -> Mux1/4
  Integrator/1 -> Mux1/6
  s/1 -> Mux1/5, Derivative/1, Integrator/1
  Derivative/1 -> Mux1/7
  myPi/1 -> Mux1/8
  Td/1 -> Mux1/9

== system adaptivePID/Adaptive PID1/y controller1/error subsystem ==
  e : Inport
  Derivative : Derivative
  Integrator : Integrator
  Mux : Mux  Inputs=3
  MyPi : Outport
  wires:
  e/1 -> Derivative/1, Mux/1, Integrator/1
  Integrator/1 -> Mux/2
  Mux/1 -> MyPi/1
  Derivative/1 -> Mux/3

== system adaptivePID/Adaptive PID1/z controller2/PID controller ==
  theta : Inport
  MyPi : Inport  Port=2
  Interpreted MATLAB Function1 : MATLABFcn  MATLABFcn=controlLaw  OutputDimensions=1
  Mux2 : Mux  Inputs=2
  u : Outport
  wires:
  Mux2/1 -> Interpreted MATLAB Function1/1
  theta/1 -> Mux2/1
  Interpreted MATLAB Function1/1 -> u/1
  MyPi/1 -> Mux2/2

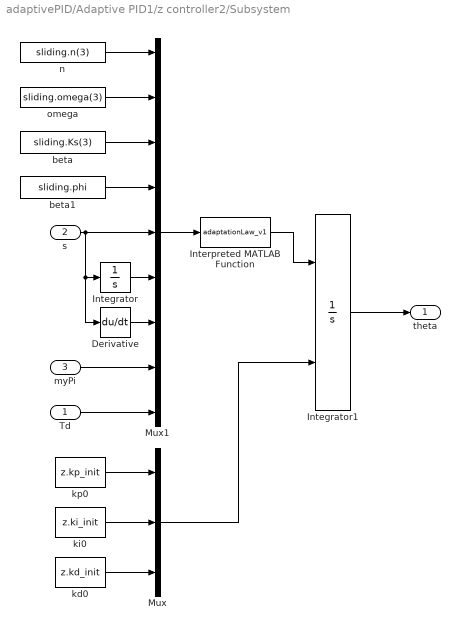
== system adaptivePID/Adaptive PID1/z controller2/Subsystem ==
  Td : Inport
  s : Inport  Port=2
  myPi : Inport  Port=3
  Derivative : Derivative
  Integrator : Integrator
  Integrator1 : Integrator  InitialConditionSource=external  InitialCondition=[1.460477259865257e-04,6.548069875818259e-05,0]
  Interpreted MATLAB Function : MATLABFcn  MATLABFcn=adaptationLaw_v1
  Mux : Mux  Inputs=3
  Mux1 : Mux  Inputs=9
  beta : Constant  Value=sliding.Ks(3)
  beta1 : Constant  Value=sliding.phi
  kd0 : Constant  Value=z.kd_init
  ki0 : Constant  Value=z.ki_init
  kp0 : Constant  Value=z.kp_init
  n : Constant  Value=sliding.n(3)
  omega : Constant  Value=sliding.omega(3)
  theta : Outport
  wires:
  beta/1 -> Mux1/3
  n/1 -> Mux1/1
  kd0/1 -> Mux/3
  kp0/1 -> Mux/1
  ki0/1 -> Mux/2
  Integrator1/1 -> theta/1
  omega/1 -> Mux1/2
  Mux1/1 -> Interpreted MATLAB Function/1
  Mux/1 -> Integrator1/2
  Interpreted MATLAB Function/1 -> Integrator1/1
  beta1/1 -> Mux1/4
  Integrator/1 -> Mux1/6
  s/1 -> Mux1/5, Derivative/1, Integrator/1
  Derivative/1 -> Mux1/7
  myPi/1 -> Mux1/8
  Td/1 -> Mux1/9

== system adaptivePID/Adaptive PID1/z controller2/error subsystem ==
  e : Inport
  Derivative : Derivative
  Integrator : Integrator
  Mux : Mux  Inputs=3
  MyPi : Outport
  wires:
  e/1 -> Derivative/1, Mux/1, Integrator/1
  Integrator/1 -> Mux/2
  Mux/1 -> MyPi/1
  Derivative/1 -> Mux/3

== matlab function adaptivePID/Subsystem1/Perturbations1 ==
  data: input input; Td output; Tb input
function Td = fcn(input, Tb)
    Lxx =  input(1);
    Rx  =  input(2);
    B_1 =  input(3);
    Lyy =  input(4);
    Ry  =  input(5);
    B_2 =  input(6);
    Lzz =  input(7);
    Rz  =  input(8);
    B_3 =  input(9);
    Lxy =  input(10);
    Lxz =  input(11);
    Lzy =  input(12);

    %%%Parameter reading
    L1 =[Lxx, (B_1/B_2)*Lxy, (B_1/B_3)*Lxz;
        (B_2/B_1)*Lxy, Lyy, (B_2/B_3)*Lzy;
        (B_3/B_1)*Lxz, (B_3/B_2)*Lzy, Lzz];
    L = [Lxx, Lxy, Lxz;
         Lxy, Lyy, Lzy;
         Lxz, Lzy, Lzz];
    R = diag([Rx,Ry,Rz]);
    B = diag([B_1,B_2,B_3]);
    
    %%% Model matrix
    Ap = -inv(L1)*R;
    Bp =  B*inv(L)*1E9; 
    Td = Ap*Tb;
end

== matlab function adaptivePID/estimator/MATLAB Function ==
  data: u input; y output
function y = fcn(u)
l = diag([u(1),u(2),u(3)]);
x = [u(4);u(5);u(6)];

y = l*x;
end

== matlab function adaptivePID/Perturbations ==
  data: u input; y output
function y = fcn(u)
y= [2.522*sin(2*pi*4.788E-3*u)+3.249E04;
   -5.174*sin(2*pi*7.481E-3*u)-2.265E04;
    3.359*sin(2*pi*8.378E-3*u)+3.655E04];
end
